simulink model "fucktrim"  (R2021b)
settings: Solver=VariableStepAuto  StartTime=0.0  StopTime=10  RelTol=1e-3
undefined symbols (not defined in the file or in its folder): drawAircraft, forces_moments, P, plotMAVStateVariables, u_trim
libraries: dspsrcs4 x1
settings Model: Creator=zhour  LastModifiedBy=zhour

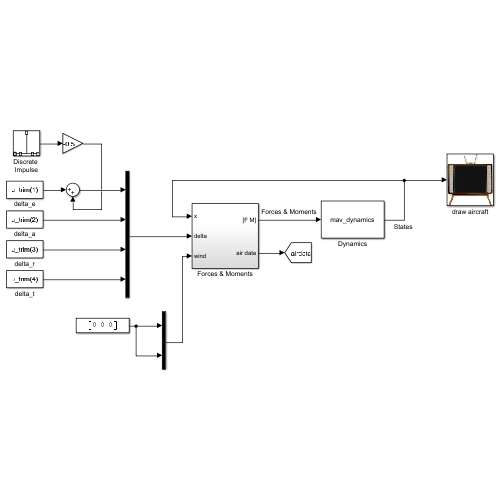
[thumbnail: Simulink's stored preview of the top-level diagram]
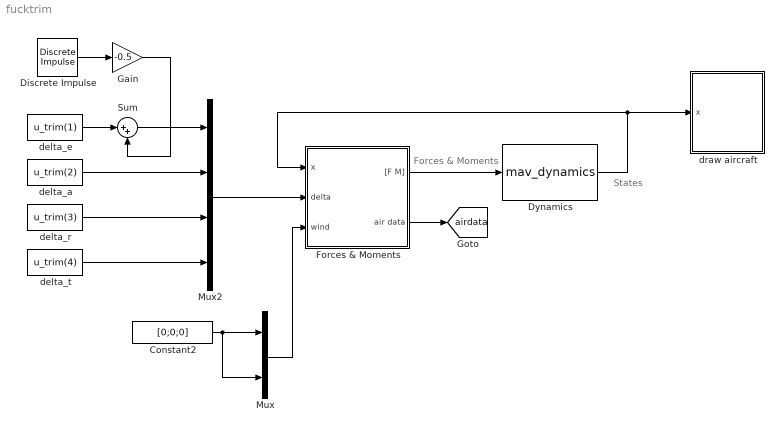
== system fucktrim ==
  note: States
  note: Forces & Moments
  Constant2 : Constant  Value=[0;0;0]
  Discrete Impulse : dspsrcs4/Discrete  Impulse  Delay=0  SampleTime=1  FrameSample=1  OutputFrames=off  dataType=double  isSigned=on  wordLen=16  udDataType=sfix(16)  fracBitsMode=Best precision  numFracBits=15  OutDataTypeStr=double  LastOutDataTypeStr=double
  Dynamics : S-Function  FunctionName=mav_dynamics  Parameters=MAV  SFunctionDeploymentMode=off  EnableBusSupport=off
  Forces & Moments : Subsystem
  Gain : Gain  Gain=-0.5
  Mux : Mux  Inputs=2
  Mux2 : Mux
  Sum : Sum  Inputs=|++
  delta_a : Constant  Value=u_trim(2)
  delta_e : Constant  Value=u_trim(1)
  delta_r : Constant  Value=u_trim(3)
  delta_t : Constant  Value=u_trim(4)
  draw aircraft : Subsystem
      mask Display: image(imread('tv.jpg'))
  tag scope: airdata=global
  wires:
  Constant2/1 -> Mux/1, Mux/2
  Forces & Moments/1("[F M]") -> Dynamics/1
  Mux2/1 -> Forces & Moments/2(delta)
  Mux/1 -> Forces & Moments/3(wind)
  Dynamics/1 -> draw aircraft/1(x), Forces & Moments/1(x)
  Forces & Moments/2(air data) -> [airdata]
  delta_a/1 -> Mux2/2
  delta_r/1 -> Mux2/3
  delta_t/1 -> Mux2/4
  delta_e/1 -> Sum/1
  Sum/1 -> Mux2/1
  Discrete Impulse/1 -> Gain/1
  Gain/1 -> Sum/2

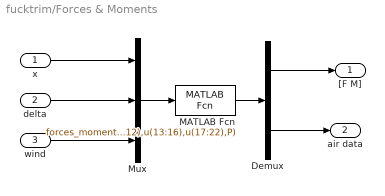
== system fucktrim/Forces & Moments ==
  x : Inport
  delta : Inport  Port=2
  wind : Inport  Port=3
  Demux : Demux  Outputs=[6;6]
  MATLAB Fcn : MATLABFcn  MATLABFcn=forces_moments(u(1:12),u(13:16),u(17:22),P)  OutputDimensions=12
  Mux : Mux  Inputs=3
  "[F M]" : Outport  VectorParamsAs1DForOutWhenUnconnected=off
  air data : Outport  Port=2  VectorParamsAs1DForOutWhenUnconnected=off
  wires:
  Demux/2 -> air data/1
  Mux/1 -> MATLAB Fcn/1
  Demux/1 -> "[F M]"/1
  MATLAB Fcn/1 -> Demux/1
  wind/1 -> Mux/3
  delta/1 -> Mux/2
  x/1 -> Mux/1

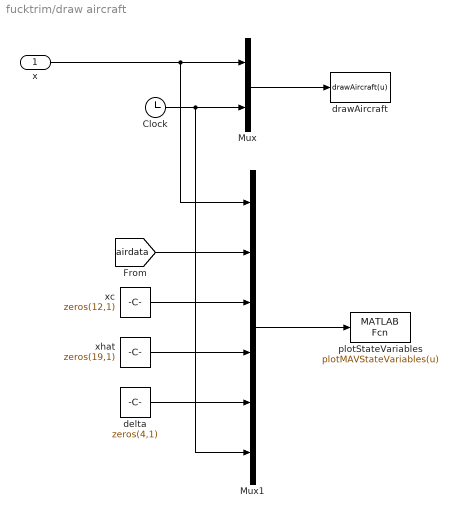
== system fucktrim/draw aircraft ==
  x : Inport
  Clock : Clock
  Mux : Mux  Inputs=2
  Mux1 : Mux  Inputs=6
  delta : Constant  Value=zeros(4,1)
  drawAircraft : MATLABFcn  MATLABFcn=drawAircraft(u)  OutputDimensions=0  SampleTime=0.1
  plotStateVariables : MATLABFcn  MATLABFcn=plotMAVStateVariables(u)  OutputDimensions=0  SampleTime=0.1
  xc : Constant  Value=zeros(12,1)
  xhat : Constant  Value=zeros(19,1)
  wires:
  [airdata] -> Mux1/2
  delta/1 -> Mux1/5
  xc/1 -> Mux1/3
  xhat/1 -> Mux1/4
  Mux1/1 -> plotStateVariables/1
  Clock/1 -> Mux1/6, Mux/2
  x/1 -> Mux1/1, Mux/1
  Mux/1 -> drawAircraft/1
